simulink model "DCMotorModel"  (R2025a)
settings: Solver=FixedStepAuto  StartTime=0.0  StopTime=10.0  RelTol=1e-3
undefined symbols (not defined in the file): kb, ki, r
settings Model: DataDictionary=Constants.sldd  Creator=levirogalla  LastModifiedBy=levirogalla

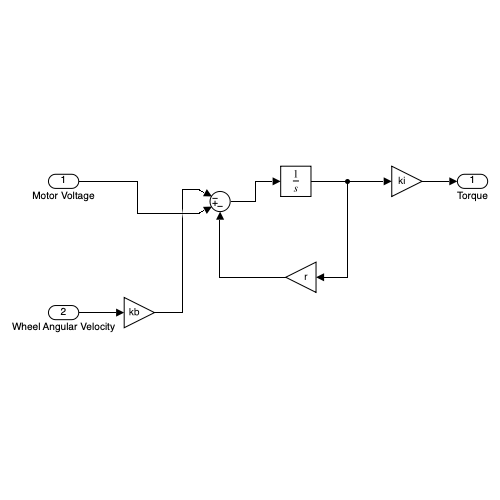
[thumbnail: Simulink's stored preview of the top-level diagram]
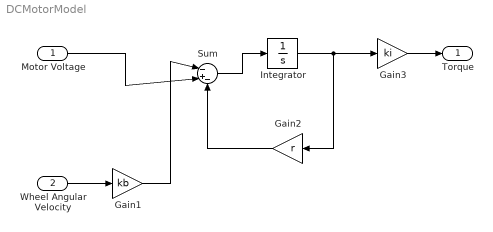
== system DCMotorModel ==
  Motor Voltage : Inport
  Wheel Angular Velocity : Inport  Port=2
  Gain1 : Gain  Gain=kb
  Gain2 : Gain  Gain=r
  Gain3 : Gain  Gain=ki
  Integrator : Integrator
  Sum : Sum  Inputs=|-+-
  Torque : Outport
  wires:
  Gain1/1 -> Sum/1
  Wheel Angular Velocity/1 -> Gain1/1
  Motor Voltage/1 -> Sum/2
  Gain3/1 -> Torque/1
  Gain2/1 -> Sum/3
  Sum/1 -> Integrator/1
  Integrator/1 -> Gain2/1, Gain3/1
